simulink model "pos_trajectory_planning"  (R2023a)
settings: configuration reference "config" (kept outside this file)
settings Model: DataDictionary=model_config.sldd  Creator=huangcheng  LastModifiedBy=Administrator
settings ConfigSetRef: SourceName=config

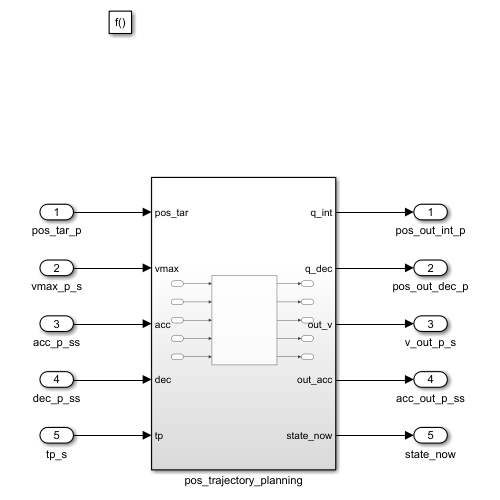
[thumbnail: Simulink's stored preview of the top-level diagram]
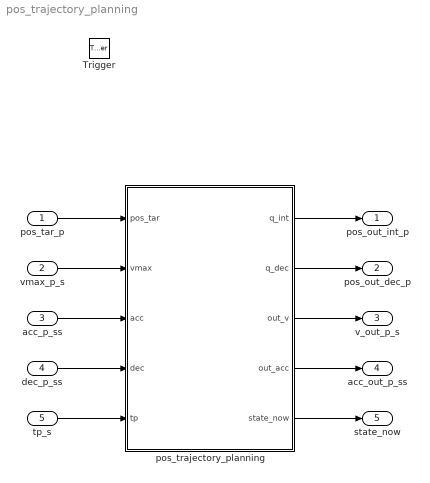
== system pos_trajectory_planning ==
  pos_tar_p : Inport  OutDataTypeStr=int64
  vmax_p_s : Inport  Port=2  OutDataTypeStr=single
  acc_p_ss : Inport  Port=3  OutDataTypeStr=single
  dec_p_ss : Inport  Port=4  OutDataTypeStr=single
  tp_s : Inport  Port=5
  Trigger : TriggerPort  TriggerType=function-call  VariantControl=(inherit)  PortDimensions=1
  pos_trajectory_planning : Subsystem
  pos_out_int_p : Outport  OutDataTypeStr=int64
  pos_out_dec_p : Outport  Port=2  OutDataTypeStr=single
  v_out_p_s : Outport  Port=3  OutDataTypeStr=single
  acc_out_p_ss : Outport  Port=4  OutDataTypeStr=single
  state_now : Outport  Port=5
  wires:
  pos_tar_p/1 -> pos_trajectory_planning/1(pos_tar)
  vmax_p_s/1 -> pos_trajectory_planning/2(vmax)
  pos_trajectory_planning/3(out_v) -> v_out_p_s/1
  acc_p_ss/1 -> pos_trajectory_planning/3(acc)
  dec_p_ss/1 -> pos_trajectory_planning/4(dec)
  tp_s/1 -> pos_trajectory_planning/5(tp)
  pos_trajectory_planning/1(q_int) -> pos_out_int_p/1
  pos_trajectory_planning/2(q_dec) -> pos_out_dec_p/1
  pos_trajectory_planning/4(out_acc) -> acc_out_p_ss/1
  pos_trajectory_planning/5(state_now) -> state_now/1

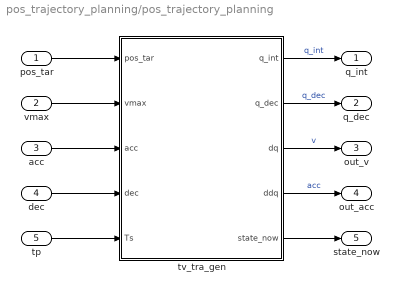
== system pos_trajectory_planning/pos_trajectory_planning ==
  pos_tar : Inport
  vmax : Inport  Port=2
  acc : Inport  Port=3
  dec : Inport  Port=4
  tp : Inport  Port=5  OutDataTypeStr=single
  tv_tra_gen : MATLAB Function
  q_int : Outport
  q_dec : Outport  Port=2
  out_v : Outport  Port=3
  out_acc : Outport  Port=4
  state_now : Outport  Port=5
  wires:
  tv_tra_gen/2(q_dec) -> q_dec/1  "q_dec"
  pos_tar/1 -> tv_tra_gen/1(pos_tar)
  vmax/1 -> tv_tra_gen/2(vmax)
  tv_tra_gen/3(dq) -> out_v/1  "v"
  acc/1 -> tv_tra_gen/3(acc)
  dec/1 -> tv_tra_gen/4(dec)
  tp/1 -> tv_tra_gen/5(Ts)
  tv_tra_gen/1(q_int) -> q_int/1  "q_int"
  tv_tra_gen/4(ddq) -> out_acc/1  "acc"
  tv_tra_gen/5(state_now) -> state_now/1

== matlab function pos_trajectory_planning/tv_tra_gen ==
  data: pos_tar input; vmax input; acc input; dec input; Ts input; q_int output; q_dec output; dq output; ddq output; state_now output
function [q_int, q_dec, dq, ddq, state_now] = tv_tra_gen(pos_tar, vmax, acc, dec, Ts)

% state_now  规划状态  
% 0 初始状态
% 1 规划完成
% 2 规划中

persistent q0_int q0_dec dq0 ddq0 state;

if isempty(q0_int)
    q0_int = int64(0);
    q0_dec = single(0);
    dq0 = single(0);
    ddq0 = single(0);
    state = int8(0);
end


vmax_abs = abs(vmax);
q1 = int64(pos_tar);
v0 = single(dq0);			 
v0_2 = v0 * v0;                   
v1 = single(0);						 
v1_2 = v1 * v1;					 
h = single(pos_tar - q0_int) - q0_dec;  %规划误差
aa = abs(acc);		 
ad = abs(dec);
aa_inv = single(0);
ad_inv = single(0);				 
vf = single(0);
Vv = single(0);
dt = Ts;
dt_inv_ = single(1.0 / dt);
Ta = single(0);
La = single(0);
Td = single(0);
Ld = single(0);
Tv = single(0);
Lv = single(0);
tt = single(0);
hd = single(1);  %误差方向

if (h >= 0)  %判断误差方向
	hd = single(1);
else
	hd = single(-1);
end

%% 轮廓速度非常小 等于 0   暂停指令会将轮廓速度设置为0
if (abs(vmax_abs) < single(0.00001))
	if (v0 > 0)
		ddq0 = -ad;
    else
		ddq0 = ad;
    end

	%根据速度判断规划完成
	if (abs(v0) < (int32(abs(ad * dt)) + int32(1)))
		dq0 = single(0);
		ddq0 = single(0);
		state = int8(1);  %规划完成
    else
        dq0 = dq0 + ddq0 * dt;
		q0_dec = q0_dec + (dq0+ single(0.5) * ddq0 * dt) * dt;
		state = int8(2);  %规划中
    end
%% 异常规划
elseif (hd * v0 < single(0))  %需要先减速到 0
	ddq0 = hd * ad;
	dq0 = dq0 + ddq0 * dt;
    q0_dec = q0_dec + (dq0+ single(0.5) * ddq0 * dt) * dt;
	state = int8(2);  %规划中
elseif (hd * v0 > vmax_abs)  %先减速到最大速度限制
	if (hd * (dq0+ (-hd * ad * dt)) <  vmax_abs)   %判断速度越界
		ddq0 = (hd * vmax_abs - v0) * dt_inv_;
		dq0 = hd * vmax_abs;
    else
		ddq0 = -hd * ad;
        dq0 = dq0 + ddq0 * dt;
    end
    q0_dec = q0_dec + (dq0+ single(0.5) * ddq0 * dt) * dt;
	state = int8(2);  %规划中
%% 正常规划
else   
	aa = hd * aa;  %加速度
	ad = -hd * ad; %减速度

	aa_inv = single(1) / aa;
	ad_inv = single(1) / ad;

	% 确定运行过程中最大速度
	kk = single(ad * aa / (ad - aa));  %运算公共系数

	% 计算运动过程中最大速度
	vf = sqrt((single(2) * h - v1_2 * ad_inv + v0_2 * aa_inv) * kk);

	vf = hd * vf;

	if (hd * vf >= vmax_abs)
		Vv = hd * vmax_abs;
    else
		Vv = vf;
    end

	% 计算加速和减速段时间
	Ta = (Vv - v0) * aa_inv;
	La = (v0 + single(0.5) * aa * Ta) * Ta;
	Td = (v1 - Vv) * ad_inv;
	Ld = (Vv + single(0.5) * ad * Td) * Td;
	Tv = (h - (Vv * Vv - v0_2) * single(0.5) * aa_inv - (v1_2 - Vv * Vv) * ...
        single(0.5) * ad_inv) / Vv;
	Lv = h - La - Ld;
	tt = dt - Ta - Tv;

	if (dt < Ta) % 加速时间
		q0_dec = q0_dec + (dq0+ single(0.5) * aa * dt) * dt;
        dq0 = dq0 + aa * dt;
		ddq0 = aa;
		state = int8(2);  %规划中
    elseif (dt >= Ta && (dt < (Ta + Tv)))  %匀速时间
        q0_dec = q0_dec + La + Vv * (dt - Ta);
		dq0 = Vv;
		ddq0 = single(0);
		state = int8(2);  %规划中
    elseif ((dt >= Ta + Tv) && (dt < Ta + Tv + Td)) % 减速时间
		pos_err = int64(pos_tar - q0_int);
		Ld_int = int64(Ld);

		if (abs(Ld_int) > abs(pos_err))  %先减速到 0
			ddq0 = ad;
            dq0 = dq0 + ddq0 * dt;
            q0_dec = q0_dec + (dq0 + single(0.5) * ddq0 * dt) * dt;
			state = int8(2);  %规划中
        else
            q0_dec = q0_dec + La + Lv + (Vv + single(0.5) * ad * tt) * tt;
            dq0 = Vv + ad * tt;
			ddq0 = ad;
			state = int8(2);  %规划中
		end
	else  %即将到达目标位置
        q0_int = q1;
        q0_dec = single(0);
		dq0 = single(0);
		ddq0 = single(0);
		state = int8(1);  %规划完成
    end
end


q0_dec_int = int64(q0_dec);

q0_dec = q0_dec - single(q0_dec_int);
q0_int = q0_int + q0_dec_int; 

q_int = q0_int;
q_dec = q0_dec;
dq = dq0;
ddq = ddq0;
state_now = state;
